simulink model "ManualLQRdesignMicroJ20F25M13wFG"  (R2025b)
settings: Solver=VariableStepAuto  StartTime=0.0  StopTime=tf  FixedStep=0.01  RelTol=1e-3
values from neighbouring files (symbols this model uses):
  Aero = struct()    [C172aeroDataM16.m]
  Deriv = struct()    [C172aeroDataM16.m]
undefined symbols (not defined in the file or in its folder): aircraft, altitudeIntegratorIC, K_lqr, K_lqr2, x_TOD, x_touchdown
libraries: simulink_extras x4, instrumentlib x3, vrlib x2, aerolibfltsims x2
settings Model: Creator=andrewbosworth  LastModifiedBy=andrewbosworth
settings DataIOCC: SaveOutput=off  SignalLogging=off  DSMLogging=off  SaveTime=off  StateSaveName=xOut  TimeSaveName=time_output  OutputSaveName=yOut

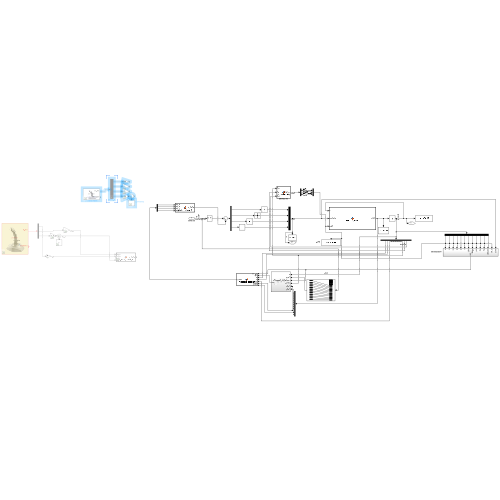
[thumbnail: Simulink's stored preview of the top-level diagram]
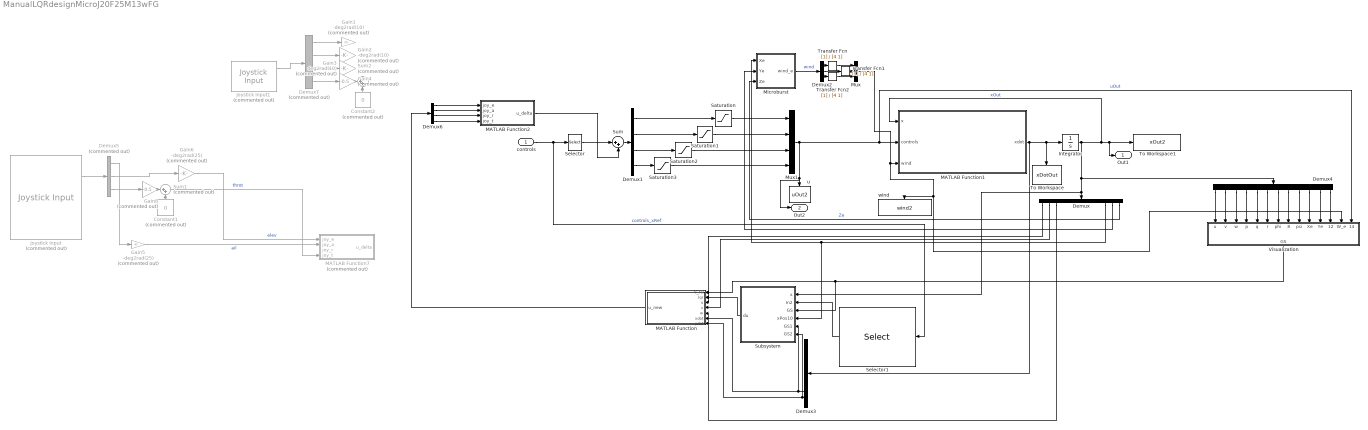
== system ManualLQRdesignMicroJ20F25M13wFG ==
  controls : Inport  PortDimensions=[16 1]
  Constant1 : Constant  Commented=on  Value=0
  Constant2 : Constant  Commented=on  Value=0
  Demux : Demux  Outputs=12
  Demux1 : Demux
  Demux2 : Demux  Outputs=3
  Demux3 : Demux  Outputs=12
  Demux4 : Demux  Outputs=12
  Demux5 : Demux  Commented=on  Outputs=3
  Demux6 : Demux
  Demux7 : Demux  Commented=on
  Gain1 : Gain  Commented=on  Gain=-deg2rad(10)
  Gain2 : Gain  Commented=on  Gain=-deg2rad(10)
  Gain3 : Gain  Commented=on  Gain=deg2rad(10)
  Gain4 : Gain  Commented=on  Gain=-0.5
  Gain5 : Gain  Commented=on  Gain=-deg2rad(25)
  Gain6 : Gain  Commented=on  Gain=-deg2rad(25)
  Gain8 : Gain  Commented=on  Gain=-0.5
  Integrator : Integrator  InitialCondition=[37.9404980038303;-0.573436414551477;2.12570252419024;0;0;0;0;0.0559687559038868;0;-6500;0;-356.623676977391]
  Joystick Input : vrlib/Joystick Input  Commented=on  joyid=1  adjustports=on  forcefeed=off
  Joystick Input1 : vrlib/Joystick Input  Commented=on  joyid=1  adjustports=on  forcefeed=off
  MATLAB Function : MATLAB Function  TreatAsAtomicUnit=on
  MATLAB Function1 : MATLAB Function  TreatAsAtomicUnit=on
  MATLAB Function2 : MATLAB Function  TreatAsAtomicUnit=on
  MATLAB Function7 : MATLAB Function  Commented=on  TreatAsAtomicUnit=on
  Microburst : MATLAB Function  TreatAsAtomicUnit=on  SystemSampleTime=0.01
  Mux : Mux  Inputs=3
  Mux1 : Mux
  Saturation : Saturate  UpperLimit=deg2rad(25)  LowerLimit=-deg2rad(25)
  Saturation1 : Saturate  UpperLimit=deg2rad(25)  LowerLimit=-deg2rad(25)
  Saturation2 : Saturate  UpperLimit=deg2rad(25)  LowerLimit=-deg2rad(25)
  Saturation3 : Saturate  UpperLimit=1  LowerLimit=0
  Selector : Selector  InputPortWidth=16  IndexOptions=Index vector (dialog)  Indices=[1 2 3 4]  OutputSizes=1
  Selector1 : Selector  InputPortWidth=16  IndexOptions=Index vector (dialog)  Indices=[5:16]  OutputSizes=1
  Subsystem : Subsystem
  Sum : Sum  Inputs=|++
  Sum1 : Sum  Commented=on  Inputs=|++
  Sum2 : Sum  Commented=on  Inputs=|++
  To Workspace : ToWorkspace  VariableName=xDotOut  SaveFormat=Timeseries  SampleTime=-1
  To Workspace1 : ToWorkspace  VariableName=xOut2  SaveFormat=Timeseries  SampleTime=-1
  Transfer Fcn : TransferFcn  Denominator=[4 1]
  Transfer Fcn1 : TransferFcn  Denominator=[4 1]
  Transfer Fcn2 : TransferFcn  Denominator=[4 1]
  Visualization : Subsystem
  u : ToWorkspace  VariableName=uOut2  SaveFormat=Timeseries  SampleTime=-1
  wind : ToWorkspace  VariableName=wind2  SaveFormat=Timeseries  SampleTime=-1
  Out1 : Outport  SignalName=x
  Out2 : Outport  Port=2  SignalName=u
  wires:
  MATLAB Function1/1(xdot) -> Demux3/1, Integrator/1, To Workspace/1
  Integrator/1 -> Out1/1, To Workspace1/1, MATLAB Function1/1(x), Demux4/1, Subsystem/1(x), Demux/1  "xOut"
  Microburst/1(wind_e) -> Demux2/1  "wind"
  Sum/1 -> Demux1/1
  Demux1/3 -> Saturation2/1
  Saturation2/1 -> Mux1/3
  Demux1/2 -> Saturation1/1
  Saturation1/1 -> Mux1/2
  Mux1/1 -> Visualization/14(uOut), MATLAB Function1/2(controls), Out2/1, u/1  "uOut"
  Demux/10 -> Subsystem/4(xPos10), Microburst/1(Xe)
  Demux/11 -> Microburst/2(Ye)
  Demux/12 -> Microburst/3(Ze)  "Ze"
  controls/1 -> Selector/1, Selector1/1  "controls_xRef"
  Selector/1 -> Sum/1
  Selector1/1 -> Subsystem/2(In2)
  Demux/1 -> MATLAB Function/3(u)
  Demux/3 -> MATLAB Function/5(w)
  Demux/2 -> MATLAB Function/4(v)
  Visualization/1(GS) -> MATLAB Function/1(V_rel), Subsystem/3(GS)
  Demux1/4 -> Saturation3/1
  Demux1/1 -> Saturation/1
  Mux/1 -> wind/1, Visualization/13(W_e), MATLAB Function1/3(wind)
  Demux2/1 -> Transfer Fcn/1
  Transfer Fcn/1 -> Mux/1
  Demux2/2 -> Transfer Fcn1/1
  Transfer Fcn1/1 -> Mux/2
  Demux2/3 -> Transfer Fcn2/1
  Transfer Fcn2/1 -> Mux/3
  Subsystem/1(du) -> MATLAB Function/2(lqr)
  Saturation3/1 -> Mux1/4
  Saturation/1 -> Mux1/1
  Demux3/11 -> Subsystem/6(GS2), MATLAB Function/7(ydot)
  Demux3/10 -> Subsystem/5(GS1), MATLAB Function/6(xdot)
  Demux4/1 -> Visualization/1(u)
  Demux4/2 -> Visualization/2(v)
  Demux4/3 -> Visualization/3(w)
  Demux4/4 -> Visualization/4(p)
  Demux4/5 -> Visualization/5(q)
  Demux4/6 -> Visualization/6(r)
  Demux4/7 -> Visualization/7(phi)
  Demux4/8 -> Visualization/8(theta)
  Demux4/9 -> Visualization/9(psi)
  Demux4/10 -> Visualization/10(Xe)
  Demux4/11 -> Visualization/11(Ye)
  Demux4/12 -> Visualization/12(altitude)
  MATLAB Function/1(u_new) -> Demux6/1
  Demux7/1 -> Gain1/1
  Demux7/3 -> Gain3/1
  Demux7/2 -> Gain2/1
  Joystick Input1/1 -> Demux7/1
  Gain4/1 -> Sum2/1
  Constant2/1 -> Sum2/2
  Demux7/4 -> Gain4/1
  Gain5/1 -> MATLAB Function7/2(joy_a)  "ail"
  Demux5/2 -> Gain6/1
  Demux5/1 -> Gain5/1
  Demux5/3 -> Gain8/1
  Joystick Input/1 -> Demux5/1
  Constant1/1 -> Sum1/2
  Gain8/1 -> Sum1/1
  Sum1/1 -> MATLAB Function7/4(joy_t)  "throt"
  Gain6/1 -> MATLAB Function7/1(joy_e)  "elev"
  Demux6/1 -> MATLAB Function2/1(joy_e)
  Demux6/2 -> MATLAB Function2/2(joy_a)
  Demux6/3 -> MATLAB Function2/3(joy_r)
  Demux6/4 -> MATLAB Function2/4(joy_t)
  MATLAB Function2/1(u_delta) -> Sum/2

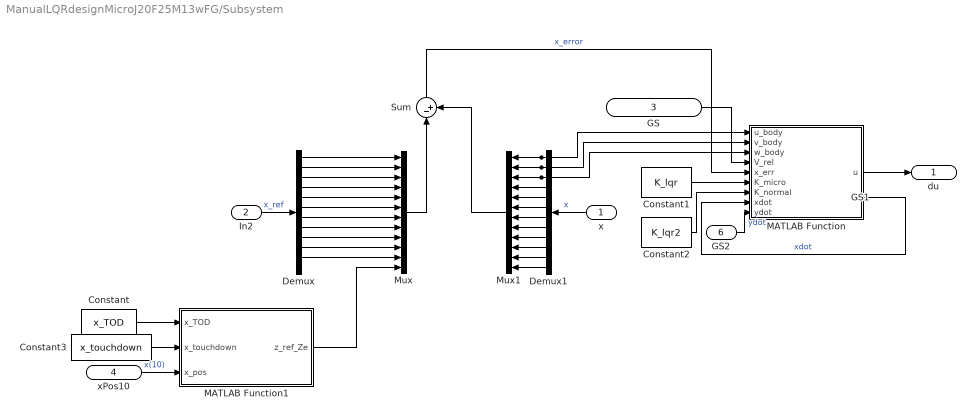
== system ManualLQRdesignMicroJ20F25M13wFG/Subsystem ==
  x : Inport
  In2 : Inport  Port=2
  GS : Inport  Port=3
  xPos10 : Inport  Port=4
  GS1 : Inport  Port=5
  GS2 : Inport  Port=6
  Constant : Constant  Value=x_TOD
  Constant1 : Constant  Value=K_lqr
  Constant2 : Constant  Value=K_lqr2
  Constant3 : Constant  Value=x_touchdown
  Demux : Demux  Outputs=12
  Demux1 : Demux  Outputs=12
  MATLAB Function : MATLAB Function  TreatAsAtomicUnit=on  SystemSampleTime=0.01
  MATLAB Function1 : MATLAB Function  TreatAsAtomicUnit=on  SystemSampleTime=0.01
  Mux : Mux  Inputs=12
  Mux1 : Mux  Inputs=12
  Sum : Sum  Inputs=|-+
  du : Outport  PortDimensions=[4 1]
  wires:
  Demux/1 -> Mux/1
  Demux/4 -> Mux/4
  Demux/5 -> Mux/5
  Demux/6 -> Mux/6
  Demux/7 -> Mux/7
  Demux/8 -> Mux/8
  In2/1 -> Demux/1  "x_ref"
  xPos10/1 -> MATLAB Function1/3(x_pos)  "x(10)"
  Demux1/1 -> Mux1/1, MATLAB Function/1(u_body)
  Demux1/2 -> Mux1/2, MATLAB Function/2(v_body)
  Demux1/3 -> Mux1/3, MATLAB Function/3(w_body)
  Demux1/4 -> Mux1/4
  Demux1/6 -> Mux1/6
  Demux1/5 -> Mux1/5
  Demux1/7 -> Mux1/7
  Demux1/8 -> Mux1/8
  Demux1/9 -> Mux1/9
  Demux1/10 -> Mux1/10
  Demux1/12 -> Mux1/12
  Demux1/11 -> Mux1/11
  x/1 -> Demux1/1  "x"
  Demux/10 -> Mux/10
  Demux/9 -> Mux/9
  GS/1 -> MATLAB Function/4(V_rel)
  Demux/2 -> Mux/2
  MATLAB Function1/1(z_ref_Ze) -> Mux/12
  Demux/3 -> Mux/3
  Sum/1 -> MATLAB Function/5(x_err)  "x_error"
  MATLAB Function/1(u) -> du/1
  Constant1/1 -> MATLAB Function/6(K_micro)
  Constant2/1 -> MATLAB Function/7(K_normal)
  Demux/11 -> Mux/11
  Mux1/1 -> Sum/2
  Mux/1 -> Sum/1
  Constant/1 -> MATLAB Function1/1(x_TOD)
  Constant3/1 -> MATLAB Function1/2(x_touchdown)
  GS1/1 -> MATLAB Function/8(xdot)  "xdot"
  GS2/1 -> MATLAB Function/9(ydot)  "ydot"

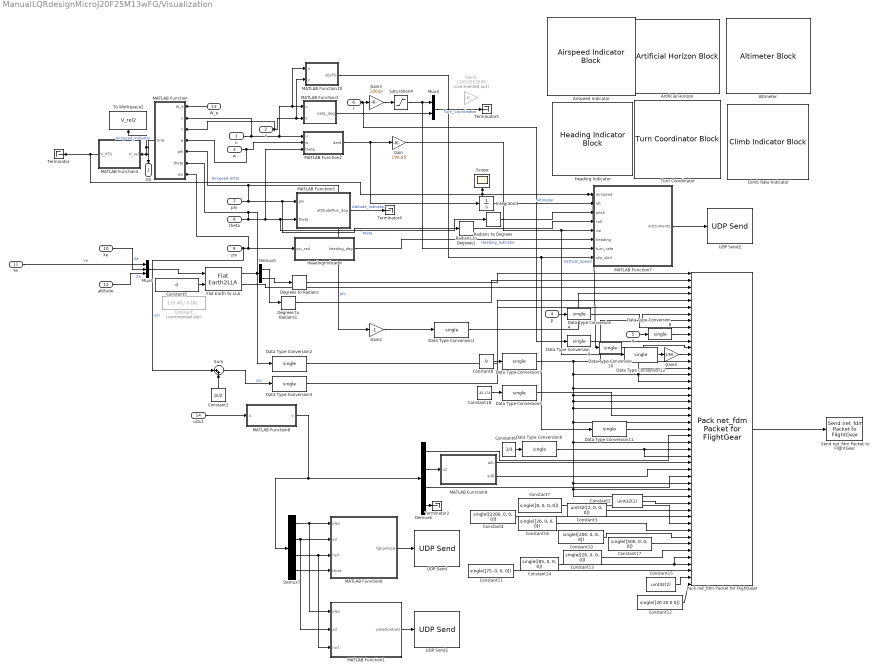
== system ManualLQRdesignMicroJ20F25M13wFG/Visualization ==
  u : Inport
  v : Inport  Port=2
  w : Inport  Port=3
  p : Inport  Port=4
  q : Inport  Port=5
  r : Inport  Port=6
  phi : Inport  Port=7
  theta : Inport  Port=8
  psi : Inport  Port=9
  Xe : Inport  Port=10
  Ye : Inport  Port=11
  altitude : Inport  Port=12
  W_e : Inport  Port=13
  uOut : Inport  Port=14
  Airspeed Indicator : AirspeedIndicatorBlock  ScaleMax=220
  Altimeter : AltimeterBlock
  Artificial Horizon : ArtificialHorizonBlock
  Climb Rate Indicator : ClimbIndicatorBlock  ScaleMax=3000
  Constant : Constant  Commented=on  Value=115.48 / 3.281
  Constant1 : Constant  Value=pi/2
  Constant10 : Constant  Value=single([200, 0, 0, 0])
  Constant11 : Constant  Value=single([75, 0, 0, 0])
  Constant12 : Constant  Value=single([20 20 0 0])
  Constant13 : Constant  Value=single([26, 0, 0, 0])
  Constant14 : Constant  Value=single([85, 0, 0, 0])
  Constant15 : Constant  Value=uint32(2)
  Constant16 : Constant  Value=single([26, 0, 0, 0])
  Constant17 : Constant  Value=single([500, 0, 0, 0])
  Constant18 : Constant  Value=-32.174
  Constant2 : Constant  Value=uint32(1)
  Constant3 : Constant  Value=uint32([2, 0, 0, 0])
  Constant4 : Constant  Value=single([2200, 0, 0, 0])
  Constant5 : Constant  Value=0
  Constant6 : Constant  Value=1/3
  Constant7 : Constant  Value=single([8, 0, 0, 0])
  Constant8 : Constant  Value=0
  Data Type Conversion{1..12} (12 alike) : DataTypeConversion  OutDataTypeStr=single  SaturateOnIntegerOverflow=off  RndMeth=Floor
  Degrees to Radians : simulink_extras/Transformations/Degrees to Radians
  Degrees to Radians1 : simulink_extras/Transformations/Degrees to Radians
  Demux5 : Demux  Outputs=2
  Demux6 : Demux
  Demux7 : Demux
  Flat Earth to LLA : FlatEarth2LLA  LL0="[40.39903955  -74.66622711]"
  Gain : Gain  Gain=196.85
  Gain1 : Gain  Commented=on  Gain=15/0.0523599
  Gain2 : Gain  Gain=-1
  Gain3 : Gain  Gain=180/pi
  Gain4 : Gain  Gain=1/60
  Heading Indicator : HeadingIndicatorBlock
  HeadingIndicator : MATLAB Function  TreatAsAtomicUnit=on
  Integrator1 : Integrator  InitialCondition=altitudeIntegratorIC
  MATLAB Function : MATLAB Function  TreatAsAtomicUnit=on
  MATLAB Function1 : MATLAB Function  TreatAsAtomicUnit=on
  MATLAB Function10 : MATLAB Function  TreatAsAtomicUnit=on
  MATLAB Function2 : MATLAB Function  TreatAsAtomicUnit=on
  MATLAB Function3 : MATLAB Function  TreatAsAtomicUnit=on
  MATLAB Function4 : MATLAB Function  TreatAsAtomicUnit=on
  MATLAB Function5 : MATLAB Function  TreatAsAtomicUnit=on
  MATLAB Function6 : MATLAB Function  TreatAsAtomicUnit=on
  MATLAB Function7 : MATLAB Function  TreatAsAtomicUnit=on
  MATLAB Function8 : MATLAB Function  TreatAsAtomicUnit=on
  MATLAB Function9 : MATLAB Function  TreatAsAtomicUnit=on
  Mux3 : Mux  Inputs=2
  Mux4 : Mux  Inputs=3
  Pack net_fdm Packet for FlightGear : aerolibfltsims/Pack net_fdm Packet for FlightGear  FlightGearVersion=v2019.1  ShowPositionAttitudeInputs=on  ShowVelocityAccelerationInputs=on  ShowControlSurfacePositionInputs=on  ShowEngineFuelInputs=on  ShowLandingGearInputs=off  ShowEnvironmentInputs=off  SampleTime=0.03  packetVersion=24
  Radians to Degrees : simulink_extras/Transformations/Radians to Degrees
  Radians to Degrees1 : simulink_extras/Transformations/Radians to Degrees
  Saturation4 : Saturate  UpperLimit=10  LowerLimit=-10
  Scope : Scope
      settings: ActiveDisplayYMinimum=-9.8114185768284514  ActiveDisplayYMaximum=154.88022552660405
  Send net_fdm Packet to FlightGear : aerolibfltsims/Send net_fdm Packet to FlightGear  DestinationIpAddress=127.0.0.1  DestinationPort=5500  LocalIpPort=-1  varLen=off  SampleTime=0.03
  Sum : Sum  Inputs=|++
  Terminator{,2,4..5} (4 alike) : Terminator
  To Workspace2 : ToWorkspace  VariableName=V_rel2  SaveFormat=Timeseries  SampleTime=-1
  Turn Coordinator : TurnCoordinatorBlock
  UDP Send : instrumentlib/UDP Send  Host=127.0.0.1  Port=5502  LocalAddress=0.0.0.0  LocalPort=-1  EnablePortSharing=off  OutputDatagramPacketSize=20  ByteOrder=big-endian  EnableBlockingMode=on  SimulateUsing=Interpreted execution
  UDP Send1 : instrumentlib/UDP Send  Host=127.0.0.1  Port=5503  LocalAddress=0.0.0.0  LocalPort=-1  EnablePortSharing=off  OutputDatagramPacketSize=20  ByteOrder=big-endian  EnableBlockingMode=on  SimulateUsing=Interpreted execution
  UDP Send2 : instrumentlib/UDP Send  Host=127.0.0.1  Port=5504  LocalAddress=0.0.0.0  LocalPort=-1  EnablePortSharing=off  OutputDatagramPacketSize=124  ByteOrder=big-endian  EnableBlockingMode=on  SimulateUsing=Interpreted execution
  GS : Outport
  wires:
  HeadingIndicator/1(heading_deg) -> MATLAB Function7/6(heading)  "Heading_Indicator"
  Gain3/1 -> Saturation4/1
  Gain/1 -> Data Type Conversion12/1, MATLAB Function7/5(vsi)  "Vertical_Speed"
  Saturation4/1 -> MATLAB Function7/7(turn_rate), Mux3/1
  Mux3/1 -> Terminator5/1  "Turn_Coordinator"
  MATLAB Function4/1(V_KTS) -> Data Type Conversion10/1, MATLAB Function7/1(airspeed), Scope/1, Terminator/1  "Airspeed (KTS)"
  MATLAB Function5/1(attitudeMux_deg) -> Terminator4/1  "Attitude_Indicator"
  MATLAB Function3/1(beta_deg) -> Mux3/2
  Integrator1/1 -> MATLAB Function7/2(alt)  "Altimeter"
  MATLAB Function/1(Vrel) -> GS/1, To Workspace2/1, MATLAB Function4/1(V_rel)  "Airspeed_Indicator"
  MATLAB Function2/1(dzdt) -> Integrator1/1, Gain/1
  MATLAB Function1/1(yokeControls) -> UDP Send1/1
  MATLAB Function6/1(fgControls) -> UDP Send/1
  Constant1/1 -> Sum/2
  psi/1 -> HeadingIndicator/1(psi_rad), MATLAB Function/7(psi), Sum/1  "psi"
  Demux6/2 -> MATLAB Function9/1(u2)
  Sum/1 -> Data Type Conversion3/1  "psi"
  Demux5/1 -> Degrees to Radians1/1
  Data Type Conversion2/1 -> Pack net_fdm Packet for FlightGear/5
  Demux7/4 -> MATLAB Function6/4(throt)
  phi/1 -> MATLAB Function/5(phi), Gain2/1, Radians to Degrees1/1, MATLAB Function5/1(phi)  "phi"
  Pack net_fdm Packet for FlightGear/1 -> Send net_fdm Packet to FlightGear/1
  Constant6/1 -> Data Type Conversion6/1
  Flat Earth to LLA/2 -> Pack net_fdm Packet for FlightGear/3
  Demux7/2 -> MATLAB Function1/2(ail), MATLAB Function6/2(ail)
  Constant8/1 -> Data Type Conversion7/1
  MATLAB Function8/1(y) -> Demux7/1, Demux6/1
  Data Type Conversion1/1 -> Pack net_fdm Packet for FlightGear/4
  Demux7/3 -> MATLAB Function1/3(rud), MATLAB Function6/3(rud)
  theta/1 -> MATLAB Function/6(theta), Data Type Conversion2/1, Radians to Degrees/1, MATLAB Function5/2(theta), MATLAB Function2/3(theta)  "theta"
  Demux7/1 -> MATLAB Function6/1(elev), MATLAB Function1/1(elev)
  Demux6/4 -> Terminator2/1
  Data Type Conversion3/1 -> Pack net_fdm Packet for FlightGear/6
  Degrees to Radians1/1 -> Pack net_fdm Packet for FlightGear/2
  Demux5/2 -> Degrees to Radians/1
  Flat Earth to LLA/1 -> Demux5/1
  Mux4/1 -> Flat Earth to LLA/1
  Constant5/1 -> Flat Earth to LLA/2
  u/1 -> MATLAB Function/2(u), MATLAB Function10/1(u), MATLAB Function3/1(u), MATLAB Function2/1(u)
  w/1 -> MATLAB Function/4(w), MATLAB Function2/2(w)
  altitude/1 -> Mux4/3  "Ze"
  W_e/1 -> MATLAB Function/1(W_e)
  uOut/1 -> MATLAB Function8/1(u)
  v/1 -> MATLAB Function10/2(v), MATLAB Function3/2(v), MATLAB Function/3(v)
  r/1 -> Data Type Conversion9/1, Gain3/1
  Xe/1 -> Mux4/2  "Xe"
  Ye/1 -> Mux4/1  "Ye"
  Radians to Degrees/1 -> MATLAB Function7/3(pitch)
  Radians to Degrees1/1 -> MATLAB Function7/4(roll)
  MATLAB Function7/1(instruments) -> UDP Send2/1
  MATLAB Function10/1(slipFG) -> Data Type Conversion11/1, MATLAB Function7/8(slip_skid)
  Data Type Conversion7/1 -> Pack net_fdm Packet for FlightGear/17, Pack net_fdm Packet for FlightGear/16, Pack net_fdm Packet for FlightGear/18, Pack net_fdm Packet for FlightGear/20, Pack net_fdm Packet for FlightGear/21, Pack net_fdm Packet for FlightGear/23, Pack net_fdm Packet for FlightGear/26, Pack net_fdm Packet for FlightGear/32, Pack net_fdm Packet for FlightGear/33, Pack net_fdm Packet for FlightGear/34, Pack net_fdm Packet for FlightGear/19, Pack net_fdm Packet for FlightGear/15, Pack net_fdm Packet for FlightGear/14, Pack net_fdm Packet for FlightGear/8, Pack net_fdm Packet for FlightGear/7
  Gain4/1 -> Pack net_fdm Packet for FlightGear/13
  Constant18/1 -> Data Type Conversion5/1
  Data Type Conversion5/1 -> Pack net_fdm Packet for FlightGear/22
  Demux6/1 -> Pack net_fdm Packet for FlightGear/25
  Data Type Conversion6/1 -> Pack net_fdm Packet for FlightGear/28, Pack net_fdm Packet for FlightGear/27
  MATLAB Function9/1(ailL) -> Pack net_fdm Packet for FlightGear/29
  MATLAB Function9/2(ailR) -> Pack net_fdm Packet for FlightGear/30
  Demux6/3 -> Pack net_fdm Packet for FlightGear/31
  Constant2/1 -> Pack net_fdm Packet for FlightGear/35
  Constant3/1 -> Pack net_fdm Packet for FlightGear/36
  Constant4/1 -> Pack net_fdm Packet for FlightGear/37
  Constant7/1 -> Pack net_fdm Packet for FlightGear/38
  Constant16/1 -> Pack net_fdm Packet for FlightGear/39
  Constant10/1 -> Pack net_fdm Packet for FlightGear/40
  Constant13/1 -> Pack net_fdm Packet for FlightGear/42
  Constant17/1 -> Pack net_fdm Packet for FlightGear/41
  Constant14/1 -> Pack net_fdm Packet for FlightGear/43, Pack net_fdm Packet for FlightGear/44
  Constant11/1 -> Pack net_fdm Packet for FlightGear/45
  Constant15/1 -> Pack net_fdm Packet for FlightGear/46
  Constant12/1 -> Pack net_fdm Packet for FlightGear/47
  p/1 -> Data Type Conversion4/1
  Data Type Conversion4/1 -> Pack net_fdm Packet for FlightGear/9
  Data Type Conversion8/1 -> Pack net_fdm Packet for FlightGear/10
  q/1 -> Data Type Conversion8/1
  Data Type Conversion9/1 -> Pack net_fdm Packet for FlightGear/11
  Data Type Conversion10/1 -> Pack net_fdm Packet for FlightGear/12
  Data Type Conversion11/1 -> Pack net_fdm Packet for FlightGear/24
  Data Type Conversion12/1 -> Gain4/1
  Degrees to Radians/1 -> Pack net_fdm Packet for FlightGear/1
  Gain2/1 -> Data Type Conversion1/1

== matlab function ManualLQRdesignMicroJ20F25M13wFG/Visualization/MATLAB Function2 ==
  data: u input; dzdt output; w input; theta input
function dzdt = dzdt(u, w, theta)
dzdt = -w*cos(theta) + u*sin(theta);
end

== matlab function ManualLQRdesignMicroJ20F25M13wFG/Visualization/MATLAB Function3 ==
  data: u input; beta_deg output; v input
function beta_deg = sideslip(u, v)
%#codegen

beta = atan2(v, u);

beta_deg = rad2deg(beta);

beta_deg = max(min(beta_deg, 15), -15);

end

== matlab function ManualLQRdesignMicroJ20F25M13wFG/Visualization/MATLAB Function4 ==
  data: V_rel input; V_KTS output
function V_KTS = vel(V_rel)

V_KTS = V_rel * 1.94384;

end

== matlab function ManualLQRdesignMicroJ20F25M13wFG/Visualization/MATLAB Function1 ==
  data: elev input; yokeControls output; ail input; rud input
% function yokeControls = normalizeYoke(elev, ail)
% %#codegen
% elev = max(min(elev / deg2rad(25), 1), -1);
% ail  = max(min(ail  / deg2rad(25), 1), -1);
% 
% % Extra safety clamp to prevent garbage values
% elev = max(min(single(elev), 1), -1);
% ail  = max(min(single(ail),  1), -1);
% 
% yokeControls = [elev, ail, elev, 0.0];
% end
% 

function yokeControls = normalizeYoke(elev, ail, rud)
%#codegen
elev = max(min(elev / deg2rad(25), 1), -1);
ail  = max(min(ail  / deg2rad(25), 1), -1);
rud  = max(min(rud  / deg2rad(25), 1), -1);

elev = max(min(single(elev), 1), -1);
ail  = max(min(single(ail),  1), -1);
rud  = max(min(single(rud),  1), -1);

% Order must match chunk order in simulink_yoke.xml:
% [yoke_elevator, yoke_aileron, yoke_elevator_norm, yoke_rudder, hide_yoke]
yokeControls = [elev, ail, elev, 0.0, -rud];
end

== matlab function ManualLQRdesignMicroJ20F25M13wFG/Visualization/MATLAB Function5 ==
  data: phi input; attitudeMux_deg output; theta input
function attitudeMux_deg = attitude(phi, theta)
%#codegen

phi_deg = max(min(rad2deg(phi), 90), -90);
theta_deg = max(min(rad2deg(theta), 30), -30);

attitudeMux_deg = [phi_deg,theta_deg];
end

== matlab function ManualLQRdesignMicroJ20F25M13wFG/Visualization/MATLAB Function10 ==
  data: u input; slipFG output; v input
function slipFG = sideslip(u, v)
%#codegen
beta = atan2(v, u);
slip = beta / deg2rad(25);  % normalize: 15 deg = full deflection
slipFG = max(min(slip, 1.0), -1.0);
end

== matlab function ManualLQRdesignMicroJ20F25M13wFG/Visualization/MATLAB Function6 ==
  data: elev input; ail input; rud input; throt input; fgControls output
function fgControls = normalizeControls(elev, ail, rud, throt)
%#codegen
% % Clamp to FG limits
elev  = max(min(elev  / deg2rad(25), 1), -1);
ail   = max(min(ail   / deg2rad(25), 1), -1);
rud   = max(min(rud   / deg2rad(25), 1), -1);
throt = max(min(throt, 1), 0);


fgControls = [elev, ail, rud, throt, throt];
end

== matlab function ManualLQRdesignMicroJ20F25M13wFG/Visualization/MATLAB Function7 ==
  data: airspeed input; instruments output; alt input; pitch input; roll input; vsi input; heading input; turn_rate input; slip_skid input
function instruments = packInstruments(airspeed, alt, pitch, roll, vsi, heading, turn_rate, slip_skid)
%#codegen
instruments = single([airspeed, alt, pitch, roll, vsi, heading, ...
    1.0, ...   % mixture full rich
    1.0, ...   % master-bat
    1.0, ...   % master-alt
    1.0, ...   % master-avionics
    3.0, ...   % magnetos both
    1.0, ...   % nav lights
    1.0, ...   % beacon
    1.0, ...   % strobe
    1.0, ...   % landing light
    1.0, ...   % taxi light
    1.0, ...   % cb master
    1.0, ...   % cb landing
    1.0, ...   % cb flaps
    0.3333, ...% flap pos norm (10 deg)
    0.3333, ...% flap lever (10 deg)
    26.5, ...  % tank0 capacity
    26.5, ...  % tank1 capacity
    12.0, ...  % tank0 level (gal)
    12.0, ...  % tank1 level (gal)
    0.0, ...   % parking brake off
    0.0, ...   % sim/model brake-parking visual
    turn_rate, ...  % turn indicator
    slip_skid, ...  % slip skid ball
    1.0, ...   % turn indicator spin (gyro up)
    1.0]);     % cb turn-coordinator
end

== matlab function ManualLQRdesignMicroJ20F25M13wFG/Visualization/MATLAB Function8 ==
  data: u input; y output
function y = normalize_inputs(u)
%#codegen
y = single(zeros(4,1));

maxRad = deg2rad(25);

y(1) = single(u(1)) / maxRad;
y(2) = - single(u(2)) / maxRad;
y(3) = single(u(3)) / maxRad;

y(4) = single(u(4));
end

== matlab function ManualLQRdesignMicroJ20F25M13wFG/Visualization/MATLAB Function9 ==
  data: u2 input; ailL output; ailR output
function [ailL, ailR] = split_aileron(u2)

ailL =  u2;   % left aileron
ailR = -u2;   % right aileron

end

== matlab function ManualLQRdesignMicroJ20F25M13wFG/MATLAB Function1 ==
  data: x input size=[12 1]; xdot output size=[12 1]; controls input; wind input; aircraft parameter; Aero parameter; Deriv parameter
function xdot = nonLinearC172(x, controls, wind, aircraft, Aero, Deriv)
%#codegen
xdot = nonLinearWindN28(x, controls, wind, Aero, Deriv, aircraft);

end

== matlab function ManualLQRdesignMicroJ20F25M13wFG/MATLAB Function2 ==
  data: joy_e input; u_delta output; joy_a input; joy_r input; joy_t input
function u_delta = joystick_clean_4(joy_e, joy_a, joy_r, joy_t)

dz_e = 0.02;
dz_a = 0.02;
dz_r = 0.04;
dz_t = 0.02;

u_delta = zeros(4,1);

u_delta(1) = apply_deadzone(joy_e, dz_e);
u_delta(2) = apply_deadzone(joy_a, dz_a);
u_delta(3) = apply_deadzone(joy_r, dz_r);
u_delta(4) = apply_deadzone(joy_t, dz_t);


% u_delta(4) = 0;
% u_delta(2) = 0;
% u_delta(3) = 0;
end


function y = apply_deadzone(x, dz)

if abs(x) < dz
    y = 0;
else
    y = sign(x) .* (abs(x) - dz) ./ (1 - dz);
end

end

== matlab function ManualLQRdesignMicroJ20F25M13wFG/MATLAB Function ==
  data: V_rel input; lqr input; u_new output; u input; v input; w input; xdot input; ydot input
function u_new = AirspeedProtection(V_rel, lqr, u, v, w, xdot, ydot)
%#codegen
% lqr = [delta_e; delta_a; delta_r; delta_t]
% V   = airspeed [m/s]

V_GS = sqrt(xdot^2 + ydot^2);

V_min = 30; % m/s

u_new = lqr;   % default: pass-through

 if (V_rel - V_GS > 15)
% if V_rel < V_min
    % Throttle: full power
    u_new(4) = 1.0;
end

% V = sqrt(u^2 + v^2 + w^2);
% 
% if abs(V_rel - V) > 1
%     % Throttle: full power
%     u_new(4) = 1.0;
% end

== matlab function ManualLQRdesignMicroJ20F25M13wFG/Subsystem/MATLAB Function ==
  data: u_body input; u output; v_body input; w_body input; V_rel input; x_err input; K_micro input; K_normal input; xdot input; ydot input
function u = lqr_blended(u_body, v_body, w_body, V_rel, x_err, K_micro, K_normal, xdot, ydot)

 V = sqrt(u_body^2 + v_body^2 + w_body^2);
%  V = sqrt(u_body^2 + v_body^2);

% V = sqrt(xdot^2 + ydot^2);

V_err = abs(V - V_rel);

V_min = 2;
V_max = 15;

alpha = (V_err - V_min) / (V_max - V_min);
alpha = max(0, min(1, alpha));

K = alpha * K_micro + (1 - alpha) * K_normal;
u = -K * x_err;
end

== matlab function ManualLQRdesignMicroJ20F25M13wFG/Microburst ==
  data: Xe input; wind_e output; Ye input; Ze input
function wind_e = MicroburstWind(Xe, Ye, Ze)
%#codegen

scaleMicroburst = 0.25;

c1 = -0.15;
c2 = -3.2175;

z_m = 394 / 3.281;    % m
u_m = 98.4 / 3.281;   % m/s
r_p = 3678.5 / 3.281; % m
alpha = 2;

% Microburst center (m)
x0 = -12000 / 3.281; 
y0 = -1000 / 3.281;

% Position
z = max(-Ze, 0);
x = Xe - x0;
y = Ye - y0;

r = sqrt(x^2 + y^2);

% Cutoff region
if r > 2.5*r_p || z > 2.5*z_m
    wind_e = [0; 0; 0];
    return;
end

% Scaling
lambda = 2*u_m / (r_p*(exp(c1)-exp(c2))*exp(1/(2*alpha)));

R = (r^(2*alpha)) / (r_p^(2*alpha));
E = exp((2 - R) / (2*alpha));

fz = exp(c1*z/z_m) - exp(c2*z/z_m);

% Radial outflow
u = lambda * x/2 * fz * E;
v = lambda * y/2 * fz * E;

% Downdraft
w = -lambda * ((z_m/c1)*(exp(c1*z/z_m)-1) ...
    - (z_m/c2)*(exp(c2*z/z_m)-1) ) * (1 - R/2) * E;

wind_e = scaleMicroburst * [u; v; w];

end

== matlab function ManualLQRdesignMicroJ20F25M13wFG/MATLAB Function7 ==
  data: joy_e input; u_delta output; joy_a input; joy_r input; joy_t input
function u_delta = joystick_clean_4(joy_e, joy_a, joy_r, joy_t)

dz_e = 0.005;
dz_a = 0.005;
dz_r = 0.04;
dz_t = 0.02;

u_delta = zeros(4,1);

u_delta(1) = apply_deadzone(joy_e, dz_e);
u_delta(2) = apply_deadzone(joy_a, dz_a);
u_delta(3) = apply_deadzone(joy_r, dz_r);
u_delta(4) = apply_deadzone(joy_t, dz_t);


% u_delta(4) = 0;
% u_delta(2) = 0;
% u_delta(3) = 0;
end


function y = apply_deadzone(x, dz)

if abs(x) < dz
    y = 0;
else
    y = sign(x) .* (abs(x) - dz) ./ (1 - dz);
end

end

== matlab function ManualLQRdesignMicroJ20F25M13wFG/Visualization/HeadingIndicator ==
  data: psi_rad input; heading_deg output
function heading_deg = wrapHeading(psi_rad)

    heading_deg = rad2deg(psi_rad);
    heading_deg = mod(heading_deg, 360);

end

== matlab function ManualLQRdesignMicroJ20F25M13wFG/Subsystem/MATLAB Function1 ==
  data: x_TOD input; x_touchdown input; x_pos input; z_ref_Ze output
% function z_ref_Ze  = glideslope_ref(x_pos)
%     z_ref_Ze = x_pos * tan(deg2rad(3));
%     z_ref_Ze = min(z_ref_Ze, 0);
% end

% function z_ref_Ze = glideslope_ref(x_pos, z_pos)
% 
%     if x_pos < (-30000 / 3.281)
%         z_ref_Ze = z_pos;
%     else
%         % 3-degree glide slope
%         z_ref_Ze = x_pos * tan(deg2rad(3));
%         z_ref_Ze = min(z_ref_Ze, 0);
%     end
% 
% end

% function z_ref_Ze = glideslope_ref(x_TOD, x_touchdown, x_pos, z_pos)
% 
%     gamma = deg2rad(3);
% 
%     blend_width = 1500;
% 
%     z_gs = (x_pos - x_touchdown) * tan(gamma);
% 
%     s = -(x_pos - x_TOD) / blend_width;
%     s = max(0, min(1, s));
% 
%    % Smooth cubic
%     s = 3*s^2 - 2*s^3;
% 
%  %   Blend
%     z_ref_Ze = (1 - s)*z_pos + s*z_gs;
% 
%   %  Stay above runway
%     z_ref_Ze = min(z_ref_Ze, 0);
% 
% end

function z_ref_Ze = glideslope_ref(x_TOD, x_touchdown, x_pos)
    gamma = deg2rad(3);
    blend_width = 1500;

    % Altitude at TOD
    z_TOD = (x_TOD - x_touchdown) * tan(gamma);
    % Glideslope from TOD
    z_gs = (x_pos - x_touchdown) * tan(gamma);

    if x_pos <= x_TOD
        z_ref_Ze = z_TOD;
    else
        % Blend from level into glideslope over blend_width
        s = (x_pos - x_TOD) / blend_width;
        s = max(0, min(1, s));
        s = 3*s^2 - 2*s^3;
        z_ref_Ze = (1 - s)*z_TOD + s*z_gs;
    end
    % Never below runway
    z_ref_Ze = min(z_ref_Ze, 0);
end

== matlab function ManualLQRdesignMicroJ20F25M13wFG/Visualization/MATLAB Function ==
  data: W_e input; u input; Vrel output; v input; w input; phi input; theta input; psi input
function Vrel = airspeed_rel(W_e,u,v,w,phi,theta,psi)
%#codegen
R = [ ...
    cos(theta)*cos(psi), cos(theta)*sin(psi), sin(theta);
    sin(phi)*sin(theta)*cos(psi)-cos(phi)*sin(psi), ...
    sin(phi)*sin(theta)*sin(psi)+cos(phi)*cos(psi), ...
    -sin(phi)*cos(theta);
    -cos(phi)*sin(theta)*cos(psi)-sin(phi)*sin(psi), ...
    -cos(phi)*sin(theta)*sin(psi)+sin(phi)*cos(psi), ...
    cos(phi)*cos(theta)];

Wb = R' * W_e(:);

u_rel = u - Wb(1);
v_rel = v - Wb(2);
w_rel = w - Wb(3);

Vrel = sqrt(u_rel^2 + v_rel^2 + w_rel^2);
end
